simulink model "ControlSystemSim"  (R2024b)
settings: Solver=VariableStepAuto  StartTime=0.0  StopTime=10.0  RelTol=1e-3
settings Model: Creator=xinxing  LastModifiedBy=xinxing

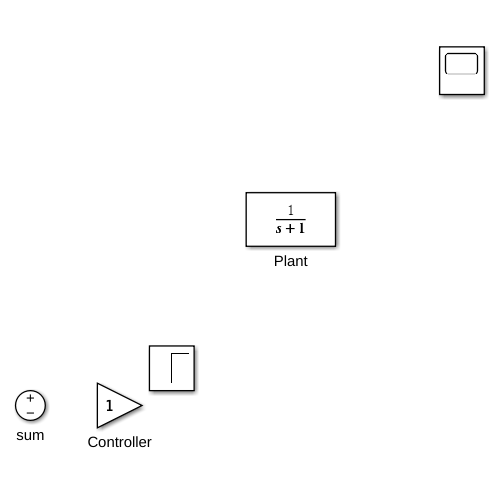
[thumbnail: Simulink's stored preview of the top-level diagram]
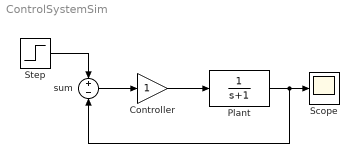
== system ControlSystemSim ==
  Controller : Gain
  Plant : TransferFcn  Denominator=[1 1]
  Scope : Scope
  Step : Step  SampleTime=0
  sum : Sum  Inputs=+-
  wires:
  Plant/1 -> Scope/1, sum/2
  Controller/1 -> Plant/1
  sum/1 -> Controller/1
  Step/1 -> sum/1
